simulink model "adc_pit_block"  (Simulink 8.8)
settings: Solver=FixedStepDiscrete  StartTime=0.0  StopTime=100.0  FixedStep=0.050  RelTol=1e-3  EnableMultiTasking=on
undefined symbols (not defined in the file or in its folder): A14, AN1, AN11, AN12, AN3, AN8, B, B13, B7, D, L3, N3, P7, PB10, PB8, PB9, PC2, PD4, PD5, PD7, PE5, R10, R4, R8, T5, U5, U7
libraries: rappid_564xl_ec_toolbox x24, simulink x4
CloseFcn:
  | rtwprivate ssgencode ModelCloseRequest tests564xl
settings Model: Creator=r61406  LastModifiedBy=eugkim01
settings SolverCC: PositivePriorityOrder=on  AutoInsertRateTranBlk=on
settings DataIOCC: ExternalInput=off  InitialState=off  LimitDataPoints=off  SaveOutput=off  SignalLogging=off  SaveTime=off
settings OptimizationCC: DefaultParameterBehavior=Inlined  EnableMemcpy=off  ExpressionDepthLimit=2147483647  InitFltsAndDblsToZero=on  LifeSpan=1
settings DebuggingCC: SolverPrmCheckMsg=warning  InheritedTsInSrcMsg=none  SingleTaskRateTransMsg=error  UnconnectedInputMsg=error  UnconnectedOutputMsg=error  UnconnectedLineMsg=error  UnknownTsInhSupMsg=error  StrictBusMsg=Warning
settings HardwareCC: ProdLargestAtomicInteger=Long  ProdLargestAtomicFloat=Double  ProdIntDivRoundTo=Zero  ProdEndianess=BigEndian  ProdHWDeviceType=Freescale->32-bit PowerPC
settings RTWCC: SystemTargetFile=rappid564xl.tlc  MakeCommand=rappid_564xl_make_rtw  TemplateMakefile=rappid_564xl_default_tmf  PostCodeGenCommand=rappid_analyzegencode(buildInfo)  Description=RAppID Toolbox MPC564xL Code Generation Target (rappid)
settings CodeAppCC: IgnoreCustomStorageClasses=off  CustomSymbolStrType=$N$R$M  InternalIdentifier=Classic
settings STFCustomTargetCC: ModelReferenceCompliant=off  IncludeMdlTerminateFcn=off  CombineOutputUpdateFcns=on  SuppressErrorStatus=on  ERTCustomFileBanners=on  SupportContinuousTime=off  SupportNonInlinedSFcns=off  RemoveResetFunc=on  MATLABClassNameForMDSCustomization=Simulink.SoftwareTarget.ERTCustomization  GRTInterface=off  SystemTargetFile=rappid564xl.tlc
settings ERTTargetCC: MultiwordLength=2048  ModelReferenceCompliant=off  ParMdlRefBuildCompliant=off  CompOptLevelCompliant=off  ConcurrentExecutionCompliant=off  IncludeMdlTerminateFcn=off  SuppressErrorStatus=on  ERTFirstTimeCompliant=off  ModelStepFunctionPrototypeControlCompliant=off  CPPClassGenCompliant=off  UseToolchainInfoCompliant=off  ExtModeMexFile=noextcomm  InlinedParameterPlacement=NonHierarchical  ERTCustomFileTemplate=example_file_process.tlc  ConvertIfToSwitch=off  SuppressUnreachableDefaultCases=off

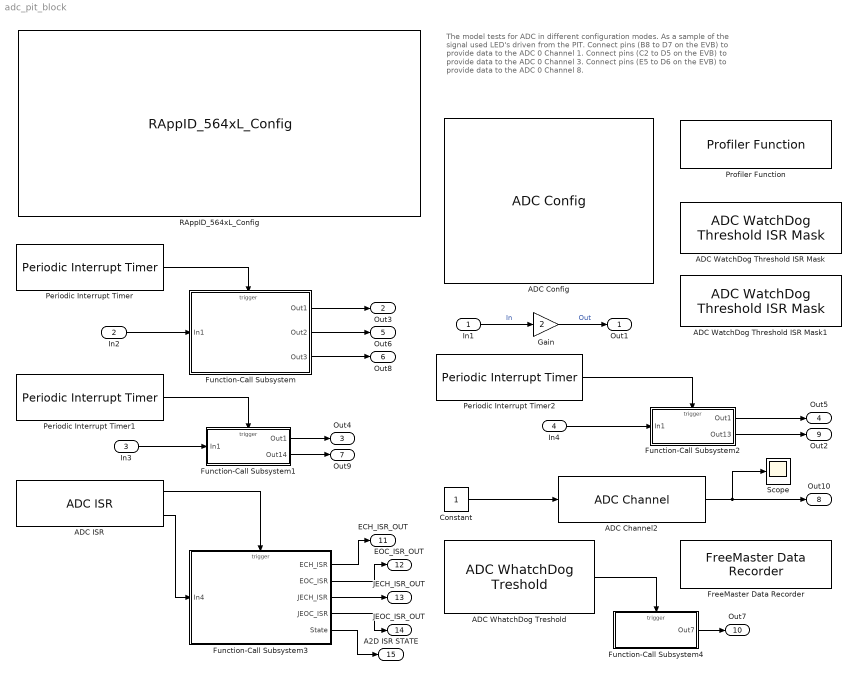
== system adc_pit_block ==
  note: The model tests for ADC in different configuration modes.
      |  As a sample of the signal used LED's driven from the PIT.
      |
      | Connect pins (B8 to D7 on the EVB) to provide data to the ADC 0 Channel 1.
      | Connect pins (C2 to D5 on the EVB) to provide data to the ADC 0 Channel 3.
      | Connect pins (E5 to D6 on the EVB) to provide data to the ADC 0 Channel 8.
  In1 : Inport
  In2 : Inport  Port=2
  In3 : Inport  Port=3
  In4 : Inport  Port=4
  ADC Channel2 : rappid_564xl_ec_toolbox/MPC564xL/Motor Control Blocks/ADC Channel  adc_unit=0  adc_chan0=older  adc_chan0_v2=69 : PE5 : [44] : [T5] : AN8  adc_chan1=older  adc_chan1_v2=26 : PB10 : [53] : [R8] : AN12  simulate=on  interrupt=on  adc_mode=Normal  adc_presample=off
  ADC Config : rappid_564xl_ec_toolbox/MPC564xL/Motor Control Blocks/ADC Config  adc_unit=0  adc_ctu=off  adc_owr=on  adc_wls=Left  adc_clk=on  adc_ack=on  adc_ctr0_inp=off  adc_ctr0_shft=10 - Avin = 0  adc_ctr0_cmp=01  adc_ctr0_samp=4  adc_ctr1_inp=off  adc_ctr1_cmp=01  adc_ctr1_samp=1  adc_ctr1_tsens=PTAT  adc_pscr_preval=V0  adc_pscr_preconv=off
  ADC ISR : rappid_564xl_ec_toolbox/MPC564xL/Motor Control Blocks/ADC ISR  adc_unit=0  adc_isr_pri=14  adc_isr_ech=off  adc_isr_eoc=off  adc_isr_jech=on  adc_isr_jeoc=on  adc_isr_eoctu=off
  ADC WatchDog Threshold ISR Mask : rappid_564xl_ec_toolbox/MPC564xL/Motor Control Blocks/ADC WatchDog Threshold ISR Mask  adc_unit=0  adc_chan0=older  adc_chan0_v2=24 : PB8 : [47] : [P7] : AN1  adc_chan1=older  adc_chan1_v2=25 : PB9 : [52] : [U7] : AN11  adc_isr_mask=Low & High Value Mask - On
  ADC WatchDog Threshold ISR Mask1 : rappid_564xl_ec_toolbox/MPC564xL/Motor Control Blocks/ADC WatchDog Threshold ISR Mask  adc_unit=0  adc_chan0=older  adc_chan0_v2=24 : PB8 : [47] : [P7] : AN1  adc_chan1=older  adc_chan1_v2=25 : PB9 : [52] : [U7] : AN11  adc_isr_mask=Low & High Value Mask - Off
  ADC WhatchDog Treshold : rappid_564xl_ec_toolbox/MPC564xL/Motor Control Blocks/ADC WhatchDog Treshold  adc_unit=0  adc_chan0=older  adc_chan0_v2=24 : PB8 : [47] : [P7] : AN1  adc_chan1=older  adc_chan1_v2=25 : PB9 : [52] : [U7] : AN11  adc_treshold=Oops  adc_treshold_value=2000  adc_up_value=2000  adc_mask_up=on  adc_low_value=800  adc_mask_low=on  adc_isr_pri=12
  Constant : Constant
  FreeMaster Data Recorder : rappid_564xl_ec_toolbox/MPC564xL/Utility Blocks/FreeMaster Data Recorder
  Function-Call Subsystem : Subsystem  TreatAsAtomicUnit=on
      settings: RTWSystemCode=Nonreusable function
  Function-Call Subsystem1 : Subsystem  TreatAsAtomicUnit=on
      settings: RTWSystemCode=Nonreusable function
  Function-Call Subsystem2 : Subsystem  TreatAsAtomicUnit=on
      settings: RTWSystemCode=Nonreusable function
  Function-Call Subsystem3 : Subsystem  TreatAsAtomicUnit=on
      settings: RTWSystemCode=Nonreusable function
  Function-Call Subsystem4 : Subsystem  TreatAsAtomicUnit=on
      settings: RTWSystemCode=Nonreusable function
  Gain : Gain  Gain=2
  Periodic Interrupt Timer : rappid_564xl_ec_toolbox/MPC564xL/General Purpose Blocks/Periodic Interrupt Timer  pit_chan=1  pit_timeout=200  int_priority=12  pit_timeout_val=23999999
  Periodic Interrupt Timer1 : rappid_564xl_ec_toolbox/MPC564xL/General Purpose Blocks/Periodic Interrupt Timer  pit_chan=2  pit_timeout=100  int_priority=12  pit_timeout_val=11999999
  Periodic Interrupt Timer2 : rappid_564xl_ec_toolbox/MPC564xL/General Purpose Blocks/Periodic Interrupt Timer  pit_chan=3  pit_timeout=250  int_priority=12  pit_timeout_val=29999999
  "Profiler Function " : rappid_564xl_ec_toolbox/MPC564xL/Utility Blocks/Profiler Function   profile_indx=1
  RAppID_564xL_Config : rappid_564xl_ec_toolbox/MPC564xL/RAppID_564xL_Config  SystemClock=120  XTAL=40  MC_clock_60=12  MC_clock_80=16  MC_clock_120=10  SWG_clock_60=20  SWG_clock_80=13.334  SWG_clock_120=20  Compiler=CodeWarrior  MemTarget=RAM  Part=MPC5643L  Package=144 LQFP  global_int_priority=10  base_tick_priority=11  sys_task_supress=off  exception_handlers=off  stored_mdl_name=rappid_564xl_ec_toolbox  freemaster_interface=Oops  freemaster_rx_pin="LINFlex_0 Rx Pin 116 : \"PB[3]\""  freemaster_tx_pin="LINFlex_0 Tx Pin 114 : \"PB[2]\""  freemaster_interface_1=Serial 0  freemaster_enable=on  freemaster_rate=57600  freemaster_tx0_pin=18 : B[2] : 114 : A14  freemaster_rx0_pin=19 : B[3] : 116 : B13  freemaster_tx1_pin=57 : D[9] : 26 : L3  freemaster_rx1_pin=29 : B[13] : 60 : R10  freemaster_can_channel=1CH  freemater_can_speed=500K  freemaster_can_msgig=0x7AA  ccp_interface=None  ccp_enable=off  ccp_can_channel=CH1 (MB 0 - 1)  ccp_can_speed=500K  ccp_can_cro_id=256  ccp_can_dto_id=257  ccp_dev_id=RappID  ccp_dev_addr=0  ccp_odt=3  ccp_daq=3  pil_enable=off  pil_bam=on  comport=1  pil_rate=57600  bam_password_def=on  bam_password=0xFEEDFACECAFEBEEF  bam_sa_cs=off  bam_start_address=0x0  bam_code_size=0x7000  cons_dspi=on  cons_can=on  cons_adc=on  cons_pwm=on  cons_ctu=on  cons_swg=on  cons_eTimer=on  cons_fm=on
  Scope : Scope
  Out1 : Outport
  Out3 : Outport  Port=2
  Out4 : Outport  Port=3
  Out5 : Outport  Port=4
  Out6 : Outport  Port=5
  Out8 : Outport  Port=6
  Out9 : Outport  Port=7
  Out10 : Outport  Port=8
  Out2 : Outport  Port=9
  Out7 : Outport  Port=10
  ECH_ISR_OUT : Outport  Port=11
  EOC_ISR_OUT : Outport  Port=12
  JECH_ISR_OUT : Outport  Port=13
  JEOC_ISR_OUT : Outport  Port=14
  A2D ISR STATE : Outport  Port=15
  wires:
  In1/1 -> Gain/1  "In"
  Gain/1 -> Out1/1  "Out"
  Function-Call Subsystem/1(Out1) -> Out3/1
  In2/1 -> Function-Call Subsystem/1(In1)
  Periodic Interrupt Timer/1 -> Function-Call Subsystem/Trigger
  Function-Call Subsystem1/1(Out1) -> Out4/1
  In3/1 -> Function-Call Subsystem1/1(In1)
  Periodic Interrupt Timer1/1 -> Function-Call Subsystem1/Trigger
  Function-Call Subsystem2/1(Out1) -> Out5/1
  In4/1 -> Function-Call Subsystem2/1(In1)
  Periodic Interrupt Timer2/1 -> Function-Call Subsystem2/Trigger
  Function-Call Subsystem/2(Out2) -> Out6/1
  Function-Call Subsystem/3(Out3) -> Out8/1
  Function-Call Subsystem1/2(Out14) -> Out9/1
  ADC Channel2/1 -> Out10/1, Scope/1
  Constant/1 -> ADC Channel2/1
  Function-Call Subsystem2/2(Out13) -> Out2/1
  ADC WhatchDog Treshold/1 -> Function-Call Subsystem4/Trigger
  Function-Call Subsystem4/1(Out7) -> Out7/1
  Function-Call Subsystem3/1(ECH_ISR) -> ECH_ISR_OUT/1
  Function-Call Subsystem3/2(EOC_ISR) -> EOC_ISR_OUT/1
  Function-Call Subsystem3/3(JECH_ISR) -> JECH_ISR_OUT/1
  Function-Call Subsystem3/4(JEOC_ISR) -> JEOC_ISR_OUT/1
  Function-Call Subsystem3/5(State) -> A2D ISR STATE/1
  ADC ISR/1 -> Function-Call Subsystem3/Trigger
  ADC ISR/2 -> Function-Call Subsystem3/1(In4)

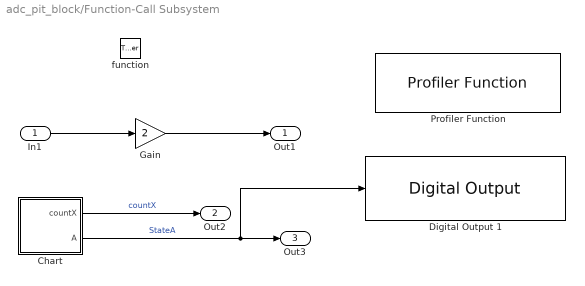
== system adc_pit_block/Function-Call Subsystem ==
  In1 : Inport
  function : TriggerPort  TriggerType=function-call  VariantControl=Variant
  Chart : Stateflow chart  TreatAsAtomicUnit=on
  Digital Output 1 : rappid_564xl_ec_toolbox/MPC564xL/General Purpose Blocks/Digital Output   gpio_outputs="52  : PD4  : [ 129 ] : [ B7 ]"  pinNum=[ 129 ]  pcrNum=52
  Gain : Gain  Gain=2
  "Profiler Function " : rappid_564xl_ec_toolbox/MPC564xL/Utility Blocks/Profiler Function   profile_indx=0
  Out1 : Outport
  Out2 : Outport  Port=2
  Out3 : Outport  Port=3
  wires:
  In1/1 -> Gain/1
  Gain/1 -> Out1/1
  Chart/1(countX) -> Out2/1  "countX"
  Chart/2(" A") -> Out3/1, Digital Output 1/1  "StateA"

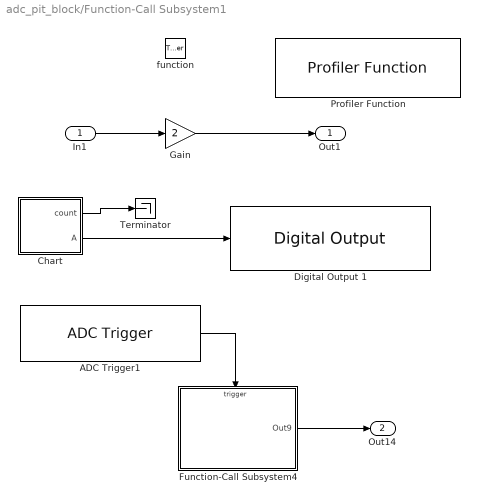
== system adc_pit_block/Function-Call Subsystem1 ==
  In1 : Inport
  function : TriggerPort  TriggerType=function-call  VariantControl=Variant
  ADC Trigger1 : rappid_564xl_ec_toolbox/MPC564xL/Motor Control Blocks/ADC Trigger  adc_unit=0  adc_mode=Normal
  Chart : Stateflow chart  TreatAsAtomicUnit=on
  Digital Output 1 : rappid_564xl_ec_toolbox/MPC564xL/General Purpose Blocks/Digital Output   gpio_outputs="53  : PD5  : [ 33 ] : [ N3 ]"  pinNum=[ 33 ]  pcrNum=53
  Function-Call Subsystem4 : Subsystem
  Gain : Gain  Gain=2
  "Profiler Function " : rappid_564xl_ec_toolbox/MPC564xL/Utility Blocks/Profiler Function   profile_indx=2
  Terminator : Terminator
  Out1 : Outport
  Out14 : Outport  Port=2
  wires:
  Gain/1 -> Out1/1
  In1/1 -> Gain/1
  Chart/2(" A") -> Digital Output 1/1
  Chart/1(count) -> Terminator/1
  ADC Trigger1/1 -> Function-Call Subsystem4/Trigger
  Function-Call Subsystem4/1(Out9) -> Out14/1

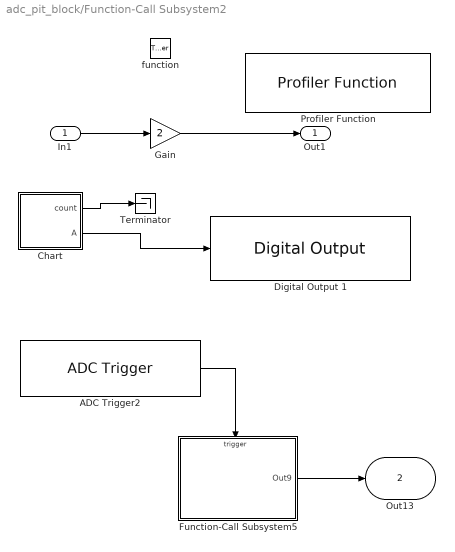
== system adc_pit_block/Function-Call Subsystem2 ==
  In1 : Inport
  function : TriggerPort  TriggerType=function-call  VariantControl=Variant
  ADC Trigger2 : rappid_564xl_ec_toolbox/MPC564xL/Motor Control Blocks/ADC Trigger  adc_unit=0  adc_mode=Injected
  Chart : Stateflow chart  TreatAsAtomicUnit=on
  Digital Output 1 : rappid_564xl_ec_toolbox/MPC564xL/General Purpose Blocks/Digital Output   gpio_outputs="55  : PD7  : [ 37 ] : [ R4 ]"  pinNum=[ 37 ]  pcrNum=55
  Function-Call Subsystem5 : Subsystem
  Gain : Gain  Gain=2
  "Profiler Function " : rappid_564xl_ec_toolbox/MPC564xL/Utility Blocks/Profiler Function   profile_indx=3
  Terminator : Terminator
  Out1 : Outport
  Out13 : Outport  Port=2
  wires:
  In1/1 -> Gain/1
  Gain/1 -> Out1/1
  Chart/2(" A") -> Digital Output 1/1
  Chart/1(count) -> Terminator/1
  ADC Trigger2/1 -> Function-Call Subsystem5/Trigger
  Function-Call Subsystem5/1(Out9) -> Out13/1

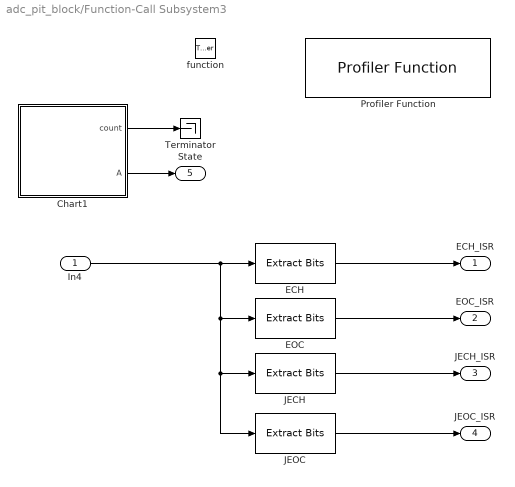
== system adc_pit_block/Function-Call Subsystem3 ==
  In4 : Inport
  function : TriggerPort  TriggerType=function-call  VariantControl=Variant
  Chart1 : Stateflow chart  TreatAsAtomicUnit=on
  ECH : simulink/Logic and Bit Operations/Extract Bits  bitsToExtract=Range of bits  numBits=8  bitIdxRange=[0]  outScalingMode=Treat bit field as an integer
  EOC : simulink/Logic and Bit Operations/Extract Bits  bitsToExtract=Range of bits  numBits=8  bitIdxRange=[1]  outScalingMode=Treat bit field as an integer
  JECH : simulink/Logic and Bit Operations/Extract Bits  bitsToExtract=Range of bits  numBits=8  bitIdxRange=[2]  outScalingMode=Treat bit field as an integer
  JEOC : simulink/Logic and Bit Operations/Extract Bits  bitsToExtract=Range of bits  numBits=8  bitIdxRange=[3]  outScalingMode=Treat bit field as an integer
  "Profiler Function " : rappid_564xl_ec_toolbox/MPC564xL/Utility Blocks/Profiler Function   profile_indx=4
  Terminator : Terminator
  ECH_ISR : Outport
  EOC_ISR : Outport  Port=2
  JECH_ISR : Outport  Port=3
  JEOC_ISR : Outport  Port=4
  State : Outport  Port=5
  wires:
  In4/1 -> ECH/1, EOC/1, JECH/1, JEOC/1
  ECH/1 -> ECH_ISR/1
  Chart1/2(" A") -> State/1
  Chart1/1(count) -> Terminator/1
  EOC/1 -> EOC_ISR/1
  JECH/1 -> JECH_ISR/1
  JEOC/1 -> JEOC_ISR/1

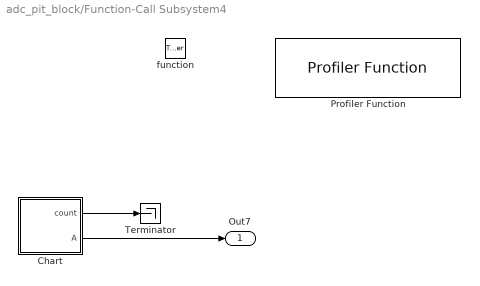
== system adc_pit_block/Function-Call Subsystem4 ==
  function : TriggerPort  TriggerType=function-call  VariantControl=Variant
  Chart : Stateflow chart  TreatAsAtomicUnit=on
  "Profiler Function " : rappid_564xl_ec_toolbox/MPC564xL/Utility Blocks/Profiler Function   profile_indx=4
  Terminator : Terminator
  Out7 : Outport
  wires:
  Chart/2(" A") -> Out7/1
  Chart/1(count) -> Terminator/1

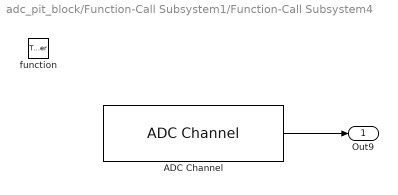
== system adc_pit_block/Function-Call Subsystem1/Function-Call Subsystem4 ==
  function : TriggerPort  TriggerType=function-call  VariantControl=Variant
  ADC Channel : rappid_564xl_ec_toolbox/MPC564xL/Motor Control Blocks/ADC Channel  adc_unit=0  adc_chan0=older  adc_chan0_v2=34 : PC2 : [45] : [U5] : AN3  adc_chan1=older  adc_chan1_v2=26 : PB10 : [53] : [R8] : AN12  simulate=off  interrupt=off  adc_mode=Normal  adc_presample=off
  Out9 : Outport
  wires:
  ADC Channel/1 -> Out9/1

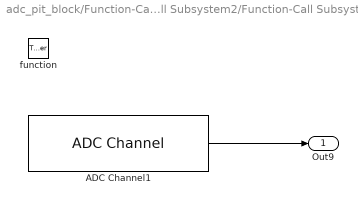
== system adc_pit_block/Function-Call Subsystem2/Function-Call Subsystem5 ==
  function : TriggerPort  TriggerType=function-call  VariantControl=Variant
  ADC Channel1 : rappid_564xl_ec_toolbox/MPC564xL/Motor Control Blocks/ADC Channel  adc_unit=0  adc_chan0=older  adc_chan0_v2=24 : PB8 : [47] : [P7] : AN1  adc_chan1=older  adc_chan1_v2=26 : PB10 : [53] : [R8] : AN12  simulate=off  interrupt=off  adc_mode=Injected  adc_presample=off
  Out9 : Outport
  wires:
  ADC Channel1/1 -> Out9/1

== stateflow chart Function-Call Subsystem4/Chart ==
  state A
  state A1
  (default) -> A : {count =0;}
  A -> A1
  A1 -> A : { count = count + 1;}
  data: count output double [0..10000]; A output boolean [0..1]

== stateflow chart Function-Call Subsystem/Chart ==
  state A
  state A1
  (default) -> A
  A -> A1
  A1 -> A : { countX = countX + 0.01;}
  data: countX output single [0..10000]; A output boolean [0..1]

== stateflow chart Function-Call Subsystem1/Chart ==
  state A
  state A1
  (default) -> A : {count =0;}
  A -> A1
  A1 -> A : { count = count + 1;}
  data: count output double [0..10000]; A output boolean [0..1]

== stateflow chart Function-Call Subsystem2/Chart ==
  state A
  state A1
  (default) -> A
  A -> A1
  A1 -> A : { count = count + 0.01;}
  data: count output double [0..10000]; A output boolean [0..1]

== stateflow chart Function-Call Subsystem3/Chart1 ==
  state A
  state A1
  (default) -> A : {count =0;}
  A -> A1
  A1 -> A : { count = count + 1;}
  data: count output double [0..10000]; A output boolean [0..1]
